simulink model "fopdt_control_PI"  (R2018a)
settings: Solver=VariableStepAuto  StartTime=0.0  StopTime=2000  MaxStep=1e-3  RelTol=1e-3
values from neighbouring files (symbols this model uses):
  kc = tau/(kp*(theta+lambda))    [Call_function.m]
  Ti = tau    [Call_function.m]
undefined symbols (not defined in the file or in its folder): DiscIntNeverNeededParam
libraries: realtime_pacer_lib x1, powerlib_meascontrol x1
settings Model: Creator=oussa  LastModifiedBy=oussa

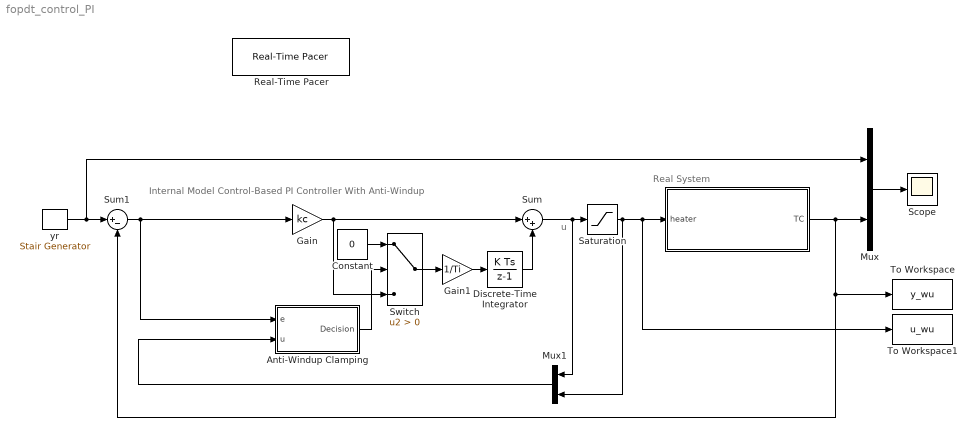
== system fopdt_control_PI ==
  note: Internal Model Control-Based PI Controller With Anti-Windup
  note: Real System
  note: u
  " " : Subsystem
  Anti-Windup Clamping : Subsystem
  Constant : Constant  Value=0
  Discrete-Time Integrator : DiscreteIntegrator  SampleTime=-1  ICPrevOutput=DiscIntNeverNeededParam  ICPrevScaledInput=DiscIntNeverNeededParam
  Gain : Gain  Gain=kc
  Gain1 : Gain  Gain=1/Ti
  Mux : Mux  Inputs=2
  Mux1 : Mux  Inputs=2
  Real-Time Pacer : realtime_pacer_lib/Real-Time Pacer  simTimePerRealTime=1
  Saturation : Saturate  UpperLimit=100  LowerLimit=0
  Scope : Scope
  Sum : Sum  Inputs=|++
  Sum1 : Sum  Inputs=|+-
  Switch : Switch  Criteria=u2 > Threshold
  To Workspace : ToWorkspace  VariableName=y_wu  SampleTime=-1
  To Workspace1 : ToWorkspace  VariableName=u_wu  SampleTime=-1
  yr : powerlib_meascontrol/Pulse & Signal Generators/Stair Generator  t=[0, 400.44, 400.45,1351.001,1351.002,2000]  e=[50,50,30,30,60,60]  Ts=0
      settings: SourceProductName=Simscape Power Systems
  wires:
  Gain1/1 -> Discrete-Time Integrator/1
  Discrete-Time Integrator/1 -> Sum/2
  " "/1(TC) -> Sum1/2, To Workspace/1, Mux/2
  Sum/1 -> Mux1/1, Saturation/1
  Saturation/1 -> To Workspace1/1, " "/1(heater), Mux1/2
  yr/1 -> Mux/1, Sum1/1
  Sum1/1 -> Gain/1, Anti-Windup Clamping/1(e)
  Gain/1 -> Switch/3, Sum/1
  Switch/1 -> Gain1/1
  Mux/1 -> Scope/1
  Constant/1 -> Switch/1
  Anti-Windup Clamping/1(Decision) -> Switch/2
  Mux1/1 -> Anti-Windup Clamping/2(u)

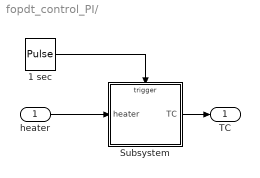
== system fopdt_control_PI/  ==
  heater : Inport  Interpolate=off
  1 sec : DiscretePulseGenerator  PulseType=Time based  Period=1  PulseWidth=50
  Subsystem : Subsystem
  TC : Outport
  wires:
  1 sec/1 -> Subsystem/Trigger
  heater/1 -> Subsystem/1(heater)
  Subsystem/1(TC) -> TC/1

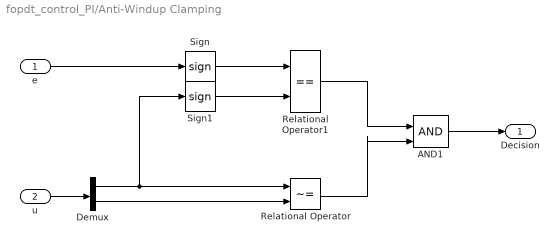
== system fopdt_control_PI/Anti-Windup Clamping ==
  e : Inport
  u : Inport  Port=2
  AND1 : Logic  IconShape=distinctive  AllPortsSameDT=off  OutDataTypeStr=boolean
  Demux : Demux  Outputs=2
  Relational Operator : RelationalOperator  Operator=~=  OutDataTypeStr=boolean  RndMeth=Simplest
  Relational Operator1 : RelationalOperator  Operator===  OutDataTypeStr=boolean  RndMeth=Simplest
  Sign : Signum
  Sign1 : Signum
  Decision : Outport
  wires:
  u/1 -> Demux/1
  e/1 -> Sign/1
  AND1/1 -> Decision/1
  Demux/1 -> Sign1/1, Relational Operator/1
  Demux/2 -> Relational Operator/2
  Sign/1 -> Relational Operator1/1
  Sign1/1 -> Relational Operator1/2
  Relational Operator/1 -> AND1/2
  Relational Operator1/1 -> AND1/1

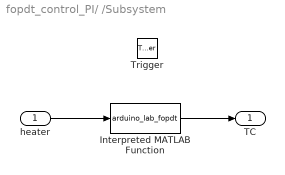
== system fopdt_control_PI/ /Subsystem ==
  heater : Inport  Interpolate=off  LatchByDelayingOutsideSignal=on
  Trigger : TriggerPort  VariantControl=Variant  PortDimensions=1
  Interpreted MATLAB Function : MATLABFcn  MATLABFcn=arduino_lab_fopdt
  TC : Outport
  wires:
  Interpreted MATLAB Function/1 -> TC/1
  heater/1 -> Interpreted MATLAB Function/1
